simulink model "prystupalab6_1_si"  (R2023b)
settings: Solver=VariableStepAuto  StartTime=0.0  StopTime=10.0  RelTol=1e-3
values from neighbouring files (symbols this model uses):
  A1 = 6    [prystupalab6.m]    (also in prystupalab6_1.m)
  A2 = 9    [prystupalab6.m]    (also in prystupalab6_1.m)
  Aw1 = 0.6    [prystupalab6.m]    (also in prystupalab6_1.m)
  Aw2 = 0.9    [prystupalab6.m]    (also in prystupalab6_1.m)
  dfw1 = 0.1*fwmax1    [prystupalab6.m]    (also in prystupalab6_1.m)
  dfw2 = 0    [prystupalab6.m]    (also in prystupalab6_1.m)
  fw1 = tabFw1(i)    [prystupalab6.m]    (also in prystupalab6_1.m)
  fw2 = 0.1*fwmax1    [prystupalab6.m]    (also in prystupalab6_1.m)
  g = 9.8    [prystupalab6.m]    (also in prystupalab6_1.m)
  H10 = (fw1^2)/(Aw1^2*2*g)    [prystupalab6_1.m]
  H20 = (fw2+fw1)^2/(Aw2^2*2*g)    [prystupalab6_1.m]
  t0 = 5    [prystupalab6.m]    (also in prystupalab6_1.m)
settings Model: Creator=Adam  LastModifiedBy=Adam

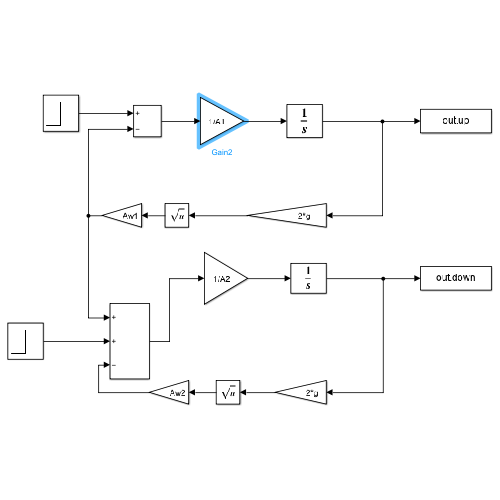
[thumbnail: Simulink's stored preview of the top-level diagram]
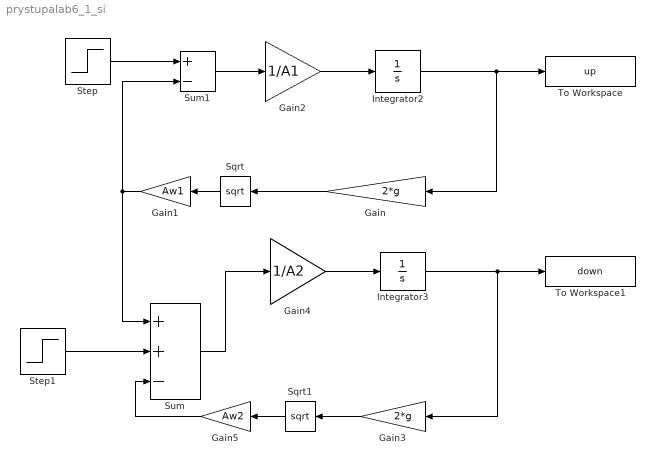
== system prystupalab6_1_si ==
  Gain : Gain  Gain=2*g
  Gain1 : Gain  Gain=Aw1
  Gain2 : Gain  Gain=1/A1
  Gain3 : Gain  Gain=2*g
  Gain4 : Gain  Gain=1/A2
  Gain5 : Gain  Gain=Aw2
  Integrator2 : Integrator  InitialCondition=H10
  Integrator3 : Integrator  InitialCondition=H20
  Sqrt : Sqrt
  Sqrt1 : Sqrt
  Step : Step  Time=t0  Before=fw1  After=fw1 + dfw1  SampleTime=0
  Step1 : Step  Time=t0  Before=fw2  After=fw2+dfw2  SampleTime=0
  Sum : Sum  Inputs=++-
  Sum1 : Sum  Inputs=+-
  To Workspace : ToWorkspace  VariableName=up  SampleTime=-1
  To Workspace1 : ToWorkspace  VariableName=down  SampleTime=-1
  wires:
  Gain3/1 -> Sqrt1/1
  Sum1/1 -> Gain2/1
  Sum/1 -> Gain4/1
  Gain2/1 -> Integrator2/1
  Step1/1 -> Sum/2
  Integrator3/1 -> Gain3/1, To Workspace1/1
  Gain4/1 -> Integrator3/1
  Integrator2/1 -> Gain/1, To Workspace/1
  Step/1 -> Sum1/1
  Sqrt/1 -> Gain1/1
  Gain/1 -> Sqrt/1
  Gain1/1 -> Sum/1, Sum1/2
  Sqrt1/1 -> Gain5/1
  Gain5/1 -> Sum/3
